simulink model "QD2_MissionCtrl_Hover_FreqSwp_2021a"  (R2026a)
settings: Solver=ode2  StopTime=inf  FixedStep=0.001  EnableMultiTasking=on
undefined symbols (not defined in the file): _MissionCtrl, datetime, Host, log_, m, qc_get_step_size, saved_data
libraries: quarc_library x29, simulink x11, simulink_extras x1
(part 1 of 2)
settings Model: SimulationMode=external  ExtModeTrigDuration=10000  Creator=Admin  LastModifiedBy=jayca
settings SolverCC: PositivePriorityOrder=on
settings RTWCC: SystemTargetFile=quarc_win64.tlc  TemplateMakefile=quarc_default_tmf  Toolchain=QUARC win64 | nmake (64-bit Windows)  BuildConfiguration=Faster Runs  Description=QUARC Win64 Target Using Toolchain
settings STFCustomTargetCC: SystemTargetFile=quarc_win64.tlc  MultiwordLength=2048.0  ConcurrentExecutionCompliant=on  UseToolchainInfoCompliant=on
settings GRTTargetCC: ExtMode=on  ExtModeMexFile=quarc_comm  ExtModeMexArgs='-w -d %d -uri %u -URI_Host tcpip://192.168.2.133:18001'  ParMdlRefBuildCompliant=off  CompOptLevelCompliant=off  CombineOutputUpdateFcns=off  MatFileLogging=off  CPPClassGenCompliant=off  GRTInterface=on

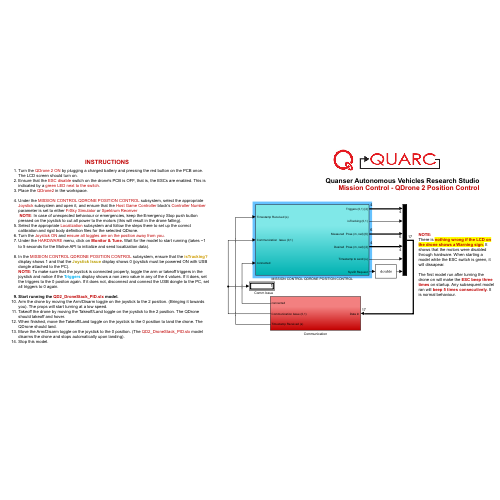
[thumbnail: Simulink's stored preview of the top-level diagram]
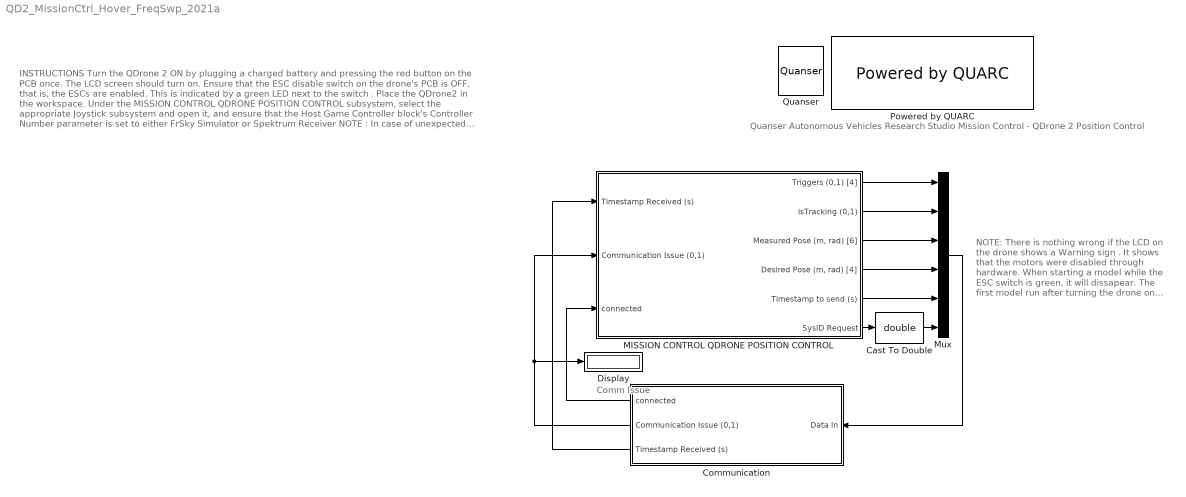
== system QD2_MissionCtrl_Hover_FreqSwp_2021a ==
  note: Quanser Autonomous Vehicles Research Studio
      | Mission Control - QDrone 2 Position Control
  note: Comm Issue
  note: INSTRUCTIONS
      |
      | Turn the QDrone 2 ON by plugging a charged battery and pressing the red button on the PCB once. The LCD screen should turn on.
      | Ensure that the ESC disable switch on the drone's PCB is OFF, that is, the ESCs are enabled. This is indicated by a green LED next to the switch .
      | Place the QDrone2 in the workspace.
      |
      | Under the MISSION CONTROL QDRONE POSITION CONTROL subsystem, select the appropriate Joystick subsystem and open it, and ensure that the Host Game Controller block's Controller Number parameter is set to either FrSky Simulator or Spektrum Receiver
      | NOTE : In case of unexpected behaviour or emergencies, keep the Emergency Stop push button pressed on the joystick to cut all power to the motors (this will result in the drone falling).
      | Select the appropriate Localization subsystem and follow the steps there to set up the correct calibration and rigid body definition files for the selected QDrone.
      | Turn the Joystick ON and ensure all toggles are on the position away from you .
      | Under the HARDWARE menu, click on Monitor & Tune . Wait for the model to start running (takes ~1 to 5 seconds for the Motive API to initialize and send localization data).
      |
      | In the MISSION CONTROL QDRONE POSITION CONTROL subsystem, ensure that the isTracking? display shows 1 and that the Joystick Issue display shows 0 (joystick must be powered ON with USB dongle attached to the PC).
      | NOTE: To make sure that the joystick is connected properly, toggle the arm or takeoff triggers in the joystick and notice if the Triggers display shows a non zero value in any of the 4 values. If it does, set the triggers to the 0 positon again. If it does not, disconnect and connect the USB dongle to the PC, set all triggers to 0 again.
      |
      | Start running the QD2_DroneStack_PID.slx model.
      | Arm the drone by moving the Arm/Disarm toggle on the joystick to the 2 position. (Bringing it towards you). The props will start turning at a low speed.
      | Takeoff the drone by moving the Takeoff/Land toggle on the joystick to the 2 position. The QDrone should takeoff and hover.
      | When finished, move the Takeoff/Land toggle on the joystick to the 0 position to land the drone. The QDrone should land.
      | Move the Arm/Disarm toggle on the joystick to the 0 position. (The QD2_DroneStack_PID.sl x model disarms the drone and stops automatically upon landing).
      | Stop this model.
  note: NOTE:
      | There is nothing wrong if the LCD on the drone shows a Warning sign . It shows that the motors were disabled through hardware. When starting a model while the ESC switch is green, it will dissapear.
      |
      | The first model run after turning the drone on will make the ESC beep three times on startup. Any subsequent model ran will beep 5 times consecutively. It is normal behaviour.
  Cast To Double : DataTypeConversion  OutDataTypeStr=double  SaturateOnIntegerOverflow=off  RndMeth=Floor
  Communication : Subsystem
  Display : Display
  MISSION CONTROL QDRONE POSITION CONTROL : Subsystem
  Mux : Mux  Inputs=6
  Powered by QUARC : quarc_library/Logos/Powered by QUARC
  Quanser : quarc_library/Logos/Quanser
  wires:
  Communication/3(Timestamp Received (s)) -> MISSION CONTROL QDRONE POSITION CONTROL/1(Timestamp Received (s))
  MISSION CONTROL QDRONE POSITION CONTROL/5(Timestamp to send (s)) -> Mux/5
  Mux/1 -> Communication/1(Data In)
  Communication/2(Communication Issue (0,1)) -> MISSION CONTROL QDRONE POSITION CONTROL/2(Communication Issue (0,1)), Display/1
  MISSION CONTROL QDRONE POSITION CONTROL/3("Measured Pose (m, rad) [6]") -> Mux/3
  MISSION CONTROL QDRONE POSITION CONTROL/4("Desired Pose (m, rad) [4]") -> Mux/4
  MISSION CONTROL QDRONE POSITION CONTROL/1(Triggers (0,1) [4]) -> Mux/1
  MISSION CONTROL QDRONE POSITION CONTROL/2(isTracking (0,1)) -> Mux/2
  Communication/1(connected) -> MISSION CONTROL QDRONE POSITION CONTROL/3(connected)
  MISSION CONTROL QDRONE POSITION CONTROL/6(SysID Request) -> Cast To Double/1
  Cast To Double/1 -> Mux/6

== system QD2_MissionCtrl_Hover_FreqSwp_2021a/Communication ==
  note: Argument (-URI_Host) is set at the MEX-file arguments
      | found at Model Configuration Properties > Code Generation > Interface
      |
      | Format:
      | tcpip://localhost:18001
  Data In : Inport
  Compare To Constant : simulink/Logic and Bit Operations/Compare To Constant  relop===  const=2  OutDataTypeStr=boolean
  Constant : Constant
  Detect Communication loss : Subsystem
  Model Argument : quarc_library/Sources/Signals/Model Argument  argument_name=URI_Host  has_value=on  data_type_mode=Specify via dialog  data_type=char  max_length=80  default_value=0  variable_size=off
      settings: AttributesFormatString=(-%<argument_name>)  SourceProductName=QUARC Targets
  Stream Server : quarc_library/Communications/Basic/Stream Server  uri_source=External input port  uri=tcpip://localhost:18877  send_buffer_size=1460  receive_buffer_size=1460  byte_order=little endian (Intel - LSB first)  optimization=Minimum latency  send_options=Send most recent data  receive_options=Receive most recent data  default_value=zeros(1,1)  sample_time=qc_get_step_size  active=off  implementation=Use blocking I/O in a separate thread  send_fifo_size=1000  receive_fifo_size=1000  send_priority=0  receive_priority=0  send_dimensions=off  receive_dimensions=off  max_dimensions=-1  data_type=Inherited via back propagation  type_expr=BusObject
  "String Display " : quarc_library/Strings/String Display  alignment=center  display_mode=Single line  sample_time=-1  use_new=off
      settings: SourceProductName=QUARC Targets
  Terminator1 : Terminator
  Terminator2 : Terminator
  connected : Outport
  Communication Issue (0,1) : Outport  Port=2  VectorParamsAs1DForOutWhenUnconnected=off
  Timestamp Received (s) : Outport  Port=3  VectorParamsAs1DForOutWhenUnconnected=off
  wires:
  Constant/1 -> Stream Server/2
  Data In/1 -> Stream Server/1
  Stream Server/3 -> Terminator2/1
  Stream Server/5 -> Terminator1/1
  Model Argument/1 -> "String Display "/1, Stream Server/3
  Stream Server/4 -> Timestamp Received (s)/1
  Stream Server/2 -> Detect Communication loss/2(Error)
  Detect Communication loss/1(Communication Issue (0,1)) -> Communication Issue (0,1)/1
  Stream Server/1 -> Compare To Constant/1, Detect Communication loss/1(State)
  Compare To Constant/1 -> connected/1

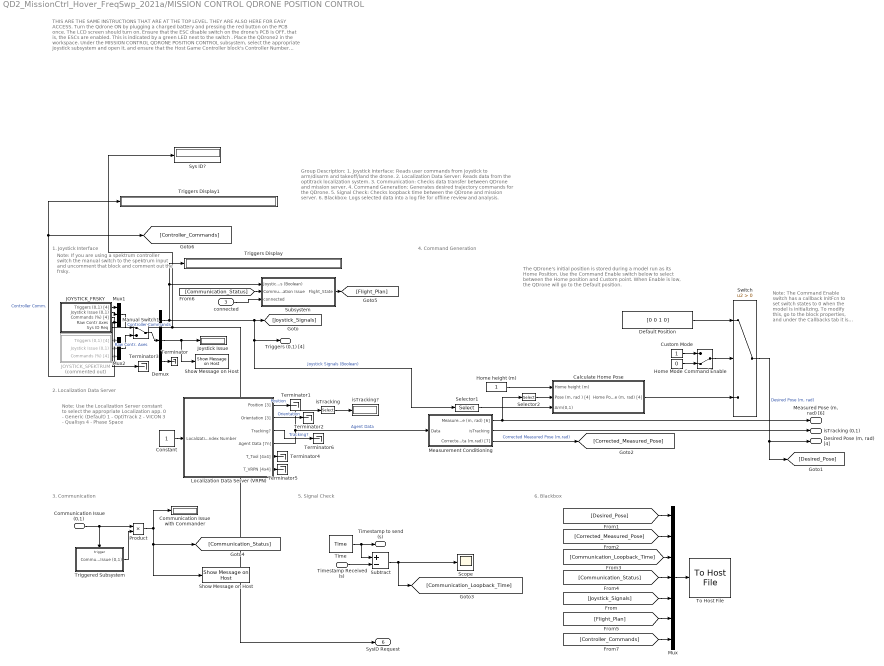
== system QD2_MissionCtrl_Hover_FreqSwp_2021a/MISSION CONTROL QDRONE POSITION CONTROL ==
  note: 5. Signal Check
  note: 6. Blackbox
  note: 3. Communication
  note: 2. Localization Data Server
  note: 1. Joystick Interface
  note: 4. Command Generation
  note: Group Description:
      |
      | 1. Joystick Interface: Reads user commands from joystick to arm/disarm and takeoff/land the drone.
      | 2. Localization Data Server: Reads data from the optitrack localization system.
      | 3. Communication: Checks data transfer between QDrone and mission server.
      | 4. Command Generation: Generates desired trajectory commands for the QDrone.
      | 5. Signal Check: Checks loopback time between the QDrone and mission server.
      | 6. Blackbox: Logs selected data into a log file for offline review and analysis.
  note: THIS ARE THE SAME INSTRUCTIONS THAT ARE AT THE TOP LEVEL. THEY ARE ALSO HERE FOR EASY ACCESS.
      |
      | Turn the Qdrone ON by plugging a charged battery and pressing the red button on the PCB once. The LCD screen should turn on.
      | Ensure that the ESC disable switch on the drone's PCB is OFF, that is, the ESCs are enabled. This is indicated by a green LED next to the switch .
      | Place the QDrone2 in the workspace.
      | Under the MISSION CONTROL QDRONE POSITION CONTROL subsystem, select the appropriate Joystick subsystem and open it, and ensure that the Host Game Controller block's Controller Number parameter is set to either FrSky Simulator or Spektrum Receiver
      | NOTE : In case of unexpected behaviour or emergencies, keep the Emergency Stop push button pressed on the joystick to cut all power to the motors (this will result in the drone falling).
      | Select the appropriate Localization subsystem and follow the steps there to set up the correct calibration and rigid body definition files for the selected QDrone.
      | Turn the Joystick ON and ensure all toggles are on the position away from you .
      | Under the HARDWARE menu, click on Monitor & Tune . Wait for the model to start running (takes ~1 to 5 seconds for the Motive API to initialize and send localization data).
      | In the MISSION CONTROL QDRONE POSITION CONTROL subsystem, ensure that the isTracking? display shows 1 and that the Joystick Issue display shows 0 (joystick must be powered ON with USB dongle attached to the PC).
      | NOTE: To make sure that the joystick is connected properly, toggle the arm or takeoff triggers in the joystick and notice if the Triggers display shows a non zero value in any of the 4 values. If it does, set the triggers to the 0 positon again. If it does not, disconnect and connect the USB dongle to the PC, set all triggers to 0 again.
      | Start running the QD2_DroneStack_PID.slx model.
      | Arm the drone by moving the Arm/Disarm toggle on the joystick to the 2 position. (Bringing it towards you). The props will start turning at a low speed.
      | Takeoff the drone by moving the Takeoff/Land toggle on the joystick to the 2 position. The QDrone should takeoff and hover.
      | When finished, move the Takeoff/Land toggle on the joystick to the 0 position to land the drone. The QDrone should land.
      | Move the Arm/Disarm toggle on the joystick to the 0 position. (The QD2_DroneStack_PID.slx model disarms the drone and stops automatically upon landing).
      | Stop this model.
  note: The QDrone's initial position is stored during a model run as its Home Position.
      | Use the Command Enable switch below to select between the Home position and Custom point. When Enable is low, the QDrone will go to the Default position.
  note: Note:
      | The Command Enable switch has a callback InitFcn to set switch states to 0 when the model is initializing. To modify this, go to the block properties, and under the Callbacks tab it is set in the InitFcn.
  note: Note:
      | If you are using a spektrum controller switch the manual switch to the spektrum input and uncomment that block and comment out the frsky.
  note: Note:
      | Use the Localization Server constant to select the appropriate Localization app.
      |
      | 0 - Generic (Default)
      | 1 - OptiTrack
      | 2 - VICON
      | 3 - Qualisys
      | 4 - Phase Space
  Timestamp Received (s) : Inport
  Communication Issue (0,1) : Inport  Port=2
  connected : Inport  Port=3
  Calculate Home Pose : Subsystem
  Command Enable : ManualSwitch  InitFcn=set_param(gcb,'sw','0')  CurrentSetting=0
  Communication Issue with Commander : Display
  Constant : Constant
  Custom Mode : Constant
  Default Position : Constant  Value=[0 0 1 0]
  Demux : Demux  Outputs=[4 1 4]
  Home Mode : Constant  Value=0
  Home height (m) : Constant
  JOYSTICK_FRSKY : Subsystem
      mask Display: image('$imagefile'); % Use "Edit Image" on toolstrip to change.
  JOYSTICK_SPEKTRUM : Subsystem  Commented=on
      mask Display: image('$imagefile'); % Use "Edit Image" on toolstrip to change.
  Joystick Issue : Display
  "Localization Data Server (VRPN) " : Subsystem
  Manual Switch1 : ManualSwitch
  Measurement Conditioning : Subsystem
  Mux : Mux  Inputs=7
  Mux1 : Mux  Inputs=[4 1 4]
  Mux2 : Mux  Inputs=[4 1 4]
  Product : Product
  Scope : Scope
      settings: ActiveDisplayYMinimum=109.87009  ActiveDisplayYMaximum=111.26511
  Selector1 : Selector  InputPortWidth=4  IndexOptions=Index vector (dialog)  Indices=[1]  OutputSizes=1
  Selector2 : Selector  InputPortWidth=6  IndexOptions=Index vector (dialog)  Indices=[1:3,6]  OutputSizes=1
  Show Message on Host : quarc_library/Sinks/Error Handling/Show Message on Host  message_type=Fixed error message  message_icon=Warning  message=Mission Control: No communication with QDrone
      settings: AttributesFormatString="\"%<message>\""  SourceProductName=QUARC Targets
  "Show Message on Host " : quarc_library/Sinks/Error Handling/Show Message on Host  message_type=Fixed error message  message_icon=Warning  message=Mission Control: Joystick Disconnected
      settings: AttributesFormatString="\"%<message>\""  SourceProductName=QUARC Targets
  Subsystem : Subsystem
  Subtract : Sum  Inputs=+-
  Switch : Switch  Criteria=u2 > Threshold  SaturateOnIntegerOverflow=off  InputSameDT=off
  Sys ID? : Display
  Terminator{,1..6} (7 alike) : Terminator
  Time : quarc_library/Sources/Time/Time  time_source=Wall clock  sample_time=qc_get_step_size
  To Host File : quarc_library/Sinks/To Host/To Host File  source=Specify via dialog (do not evaluate)  file_name=saved_data/%m/log_%{regexprep(char(datetime),' ','_')}_MissionCtrl.mat  variable_name=mission_server_data  decimation=1  sample_time=-1  file_format=MAT-file v.5  options=No header or footer  append=off  final_file_name=saved_data/QD2_MissionCtrl_Hover_FreqSwp_2021a/log_2026-09-15_19-51-03_MissionCtrl.mat  encoding=Default  bitrate=2000000
  Triggered Subsystem : Subsystem  TreatAsAtomicUnit=on
  Triggers Display : Display
  Triggers Display1 : Display
  isTracking : Selector  InputPortWidth=7  IndexOptions=Index vector (dialog)  Indices=[7]  OutputSizes=1
  isTracking? : Display
  Triggers (0,1) [4] : Outport  VectorParamsAs1DForOutWhenUnconnected=off
  isTracking (0,1) : Outport  Port=2  VectorParamsAs1DForOutWhenUnconnected=off
  "Measured Pose (m, rad) [6]" : Outport  Port=3  VectorParamsAs1DForOutWhenUnconnected=off
  "Desired Pose (m, rad) [4]" : Outport  Port=4  VectorParamsAs1DForOutWhenUnconnected=off
  Timestamp to send (s) : Outport  Port=5  VectorParamsAs1DForOutWhenUnconnected=off
  SysID Request : Outport  Port=6
  wires:
  Communication Issue (0,1)/1 -> Product/1, Triggered Subsystem/Trigger
  isTracking/1 -> isTracking?/1
  Demux/2 -> "Show Message on Host "/1, Joystick Issue/1
  Demux/3 -> Terminator/1
  Demux/1 -> Subsystem/1(Joystick Signals (Boolean)), Triggers Display/1, Selector1/1, Triggers (0,1) [4]/1, [Joystick_Signals]  "Joystick Signals (Boolean)"
  Time/1 -> Subtract/1, Timestamp to send (s)/1
  Timestamp Received (s)/1 -> Subtract/2
  Subtract/1 -> Scope/1, [Communication_Loopback_Time]
  Switch/1 -> [Desired_Pose], "Desired Pose (m, rad) [4]"/1  "Desired Pose (m, rad)"
  Measurement Conditioning/2(isTracking) -> isTracking (0,1)/1
  Calculate Home Pose/1("Home Pose (m, rad) [4]") -> Switch/3
  Home height (m)/1 -> Calculate Home Pose/1(Home height (m))
  Triggered Subsystem/1(Communication Issue (0,1)) -> Product/2
  Mux/1 -> To Host File/1
  Selector1/1 -> Calculate Home Pose/3(Arm(0,1))
  Measurement Conditioning/1("Measured Pose (m, rad) [6]") -> "Measured Pose (m, rad) [6]"/1, Selector2/1
  Measurement Conditioning/3(Corrected Pose Data (m,rad) [7]) -> [Corrected_Measured_Pose]  "Corrected Measured Pose (m,rad)"
  JOYSTICK_SPEKTRUM/1(Triggers (0,1) [4]) -> Mux2/1
  JOYSTICK_SPEKTRUM/2(Joystick Issue (0,1)) -> Mux2/2
  JOYSTICK_SPEKTRUM/3(Commands (%) [4]) -> Mux2/3
  Manual Switch1/1 -> Demux/1
  Mux2/1 -> Manual Switch1/2
  Home Mode/1 -> Command Enable/2
  Custom Mode/1 -> Command Enable/1
  Command Enable/1 -> Switch/2
  JOYSTICK_FRSKY/2(Joystick Issue (0,1)) -> Mux1/2
  JOYSTICK_FRSKY/1(Triggers (0,1) [4]) -> Mux1/1
  JOYSTICK_FRSKY/3(Commands (%) [4]) -> Triggers Display1/1, [Controller_Commands], Mux1/3  "Controller Comm."
  Mux1/1 -> Manual Switch1/1  "Controller Commands"
  "Localization Data Server (VRPN) "/4(Agent Data [7n]) -> isTracking/1, Measurement Conditioning/1(Data)  "Agent Data"
  Selector2/1 -> Calculate Home Pose/2("Pose (m, rad ) [4]")
  [Joystick_Signals] -> Mux/5
  [Desired_Pose] -> Mux/1
  [Corrected_Measured_Pose] -> Mux/2
  [Communication_Loopback_Time] -> Mux/3
  [Communication_Status] -> Mux/4
  Subsystem/1(Flight_State) -> [Flight_Plan]
  [Flight_Plan] -> Mux/6
  [Communication_Status] -> Subsystem/2("Communication Issue ")
  Product/1 -> Communication Issue with Commander/1, [Communication_Status], Show Message on Host/1
  Default Position/1 -> Switch/1
  connected/1 -> Subsystem/3(connected)
  Constant/1 -> "Localization Data Server (VRPN) "/1(Localization System Index Number)
  "Localization Data Server (VRPN) "/5(T_Tool [4x4]) -> Terminator4/1
  "Localization Data Server (VRPN) "/6(T_VRPN [4x4]) -> Terminator5/1
  [Controller_Commands] -> Mux/7
  "Localization Data Server (VRPN) "/1(Position [3]) -> Terminator1/1  "Position"
  "Localization Data Server (VRPN) "/2(Orientation [3]) -> Terminator2/1  "Orientation"
  "Localization Data Server (VRPN) "/3(Tracking?) -> Terminator6/1  "Tracking?"
  JOYSTICK_FRSKY/4(Raw Contr Axes) -> Terminator3/1  "Raw Contr. Axes"
  JOYSTICK_FRSKY/5(Sys ID Req) -> Sys ID?/1, SysID Request/1

== system QD2_MissionCtrl_Hover_FreqSwp_2021a/Communication/Detect Communication loss ==
  note: Check if stream is 2 (connected) and error is positive (error codes are negative). Otherwise issue a communication error.
  State : Inport
  Error : Inport  Port=2
  Data Type Conversion : DataTypeConversion  SaturateOnIntegerOverflow=off  RndMeth=Floor
  MATLAB Function : MATLAB Function  TreatAsAtomicUnit=on
  Terminator2 : Terminator
  Threshold : quarc_library/Discontinuities/Threshold  operator=>=  param_src=Specify via dialog  threshold=0.5  duration=0.1
      settings: SourceProductName=QUARC Targets
  Time : quarc_library/Sources/Time/Time  time_source=Wall clock  sample_time=qc_get_step_size
  Communication Issue (0,1) : Outport  VectorParamsAs1DForOutWhenUnconnected=off
  wires:
  Error/1 -> MATLAB Function/3(error)
  MATLAB Function/1(stream_connection_loss) -> Threshold/1
  State/1 -> MATLAB Function/2(state)
  Time/1 -> MATLAB Function/1(time)
  Threshold/2 -> Terminator2/1
  Data Type Conversion/1 -> Communication Issue (0,1)/1
  Threshold/1 -> Data Type Conversion/1

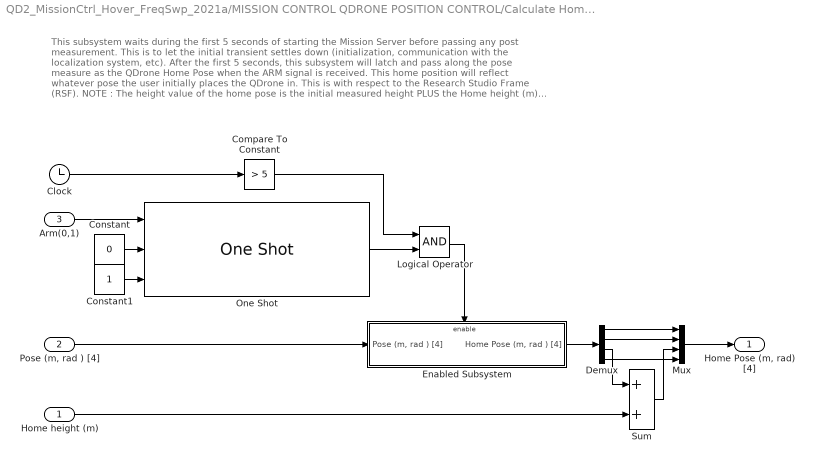
== system QD2_MissionCtrl_Hover_FreqSwp_2021a/MISSION CONTROL QDRONE POSITION CONTROL/Calculate Home Pose ==
  note: This subsystem waits during the first 5 seconds of starting the Mission Server before passing any post measurement.
      | This is to let the initial transient settles down (initialization, communication with the localization system, etc).
      | After the first 5 seconds, this subsystem will latch and pass along the pose measure as the QDrone Home Pose when
      | the ARM signal is received.
      | This home position will reflect whatever pose the user initially places the QDrone in.
      | This is with respect to the Research Studio Frame (RSF).
      |
      | NOTE : The height value of the home pose is the initial measured height PLUS the Home height (m) input value.
  Home height (m) : Inport
  "Pose (m, rad ) [4]" : Inport  Port=2
  Arm(0,1) : Inport  Port=3
  Clock : Clock
  Compare To Constant : simulink/Logic and Bit Operations/Compare To Constant  relop=>  const=5  OutDataTypeStr=boolean
  Constant : Constant  Value=0
  Constant1 : Constant
  Demux : Demux
  Enabled Subsystem : Subsystem  TreatAsAtomicUnit=on
  Logical Operator : Logic  AllPortsSameDT=off  OutDataTypeStr=boolean
  Mux : Mux
  One Shot : quarc_library/Discontinuities/One Shot  trigger_type=Rising edge  redun_pulse=Ignore extraneous pulse  width_source=Specify via dialog  pulse_width=1/qc_get_step_size
      settings: SourceProductName=QUARC Targets
  Sum : Sum
  "Home Pose (m, rad) [4]" : Outport  VectorParamsAs1DForOutWhenUnconnected=off
  wires:
  Constant/1 -> One Shot/2
  Constant1/1 -> One Shot/3
  Arm(0,1)/1 -> One Shot/1
  One Shot/1 -> Logical Operator/2
  "Pose (m, rad ) [4]"/1 -> Enabled Subsystem/1("Pose (m, rad ) [4] ")
  Clock/1 -> Compare To Constant/1
  Compare To Constant/1 -> Logical Operator/1
  Logical Operator/1 -> Enabled Subsystem/Enable
  Enabled Subsystem/1("Home Pose (m, rad ) [4]") -> Demux/1
  Demux/1 -> Mux/1
  Demux/2 -> Mux/2
  Demux/4 -> Mux/4
  Demux/3 -> Sum/1
  Sum/1 -> Mux/3
  Home height (m)/1 -> Sum/2
  Mux/1 -> "Home Pose (m, rad) [4]"/1

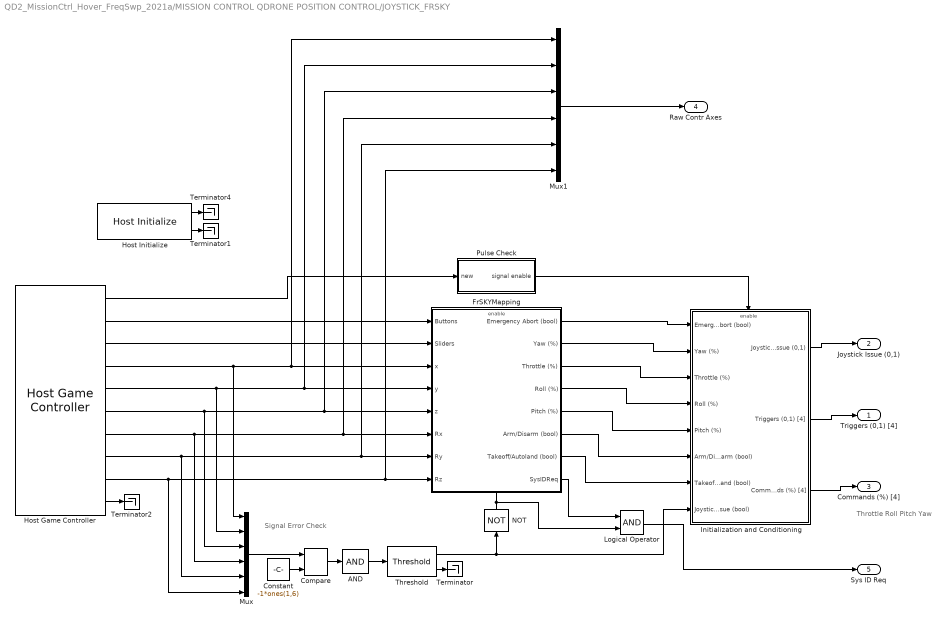
== system QD2_MissionCtrl_Hover_FreqSwp_2021a/MISSION CONTROL QDRONE POSITION CONTROL/JOYSTICK_FRSKY ==
  note: Throttle
      | Roll
      | Pitch
      | Yaw
  note: Signal Error Check
  AND : Logic  Inputs=1  AllPortsSameDT=off  OutDataTypeStr=boolean
  Compare : quarc_library/Logic Operations/Compare  operator===  output_data_type=boolean
      settings: SourceProductName=QUARC Targets
  Constant : Constant  Value=-1*ones(1,6)
  FrSKYMapping : Subsystem
  Host Game Controller : quarc_library/Devices/Peripherals/Host/Host Game Controller  object_name=Host-1  controller=1  buffer_size=20  deadzone=[]  saturation=[]  sample_time=qc_get_step_size  auto_center=off  enabled=on  debug_mode=off
      settings: SourceProductName=QUARC Targets
  Host Initialize : quarc_library/Devices/Peripherals/Host/Host Initialize  object_name=Host-1  uri_source=Use external mode communications  uri=tcpip://localhost:18001  send_buffer_size=1000  receive_buffer_size=1000  thread_priority=0  run_client=on  use_window=off  window_position=[]  sample_time=qc_get_step_size  active=on
      settings: SourceProductName=QUARC Targets
  Initialization and Conditioning : Subsystem  TreatAsAtomicUnit=on
  Logical Operator : Logic  AllPortsSameDT=off  OutDataTypeStr=boolean
  Mux : Mux  Inputs=6
  Mux1 : Mux  Inputs=6
  NOT : Logic  Operator=NOT  IconShape=distinctive  AllPortsSameDT=off  OutDataTypeStr=boolean
  Pulse Check : Subsystem  TreatAsAtomicUnit=on
  Terminator{,1..2,4} (4 alike) : Terminator
  Threshold : quarc_library/Discontinuities/Threshold  operator=>=  param_src=Specify via dialog  threshold=0.5  duration=0.2
      settings: SourceProductName=QUARC Targets
  Triggers (0,1) [4] : Outport  VectorParamsAs1DForOutWhenUnconnected=off
  Joystick Issue (0,1) : Outport  Port=2  VectorParamsAs1DForOutWhenUnconnected=off
  Commands (%) [4] : Outport  Port=3  VectorParamsAs1DForOutWhenUnconnected=off
  Raw Contr Axes : Outport  Port=4
  Sys ID Req : Outport  Port=5
  wires:
  Host Game Controller/10 -> Terminator2/1
  Pulse Check/1(signal enable) -> Initialization and Conditioning/Enable
  Host Initialize/1 -> Terminator4/1
  FrSKYMapping/6("Arm/Disarm (bool) ") -> Initialization and Conditioning/6(Arm/Disarm (bool))
  Host Initialize/2 -> Terminator1/1
  FrSKYMapping/7(Takeoff/Autoland (bool)) -> Initialization and Conditioning/7(Takeoff/AutoLand (bool))
  Host Game Controller/7 -> Mux/4, Mux1/4, FrSKYMapping/6(Rx)
  Host Game Controller/8 -> Mux/5, Mux1/5, FrSKYMapping/7(Ry)
  Initialization and Conditioning/3(Commands (%) [4]) -> Commands (%) [4]/1
  Host Game Controller/5 -> Mux/2, Mux1/2, FrSKYMapping/4(y)
  Host Game Controller/9 -> Mux/6, Mux1/6, FrSKYMapping/8(Rz)
  Host Game Controller/1 -> Pulse Check/1(new)
  Mux/1 -> Compare/1
  Threshold/1 -> NOT/1, Initialization and Conditioning/8(Joystick Issue (bool))
  AND/1 -> Threshold/1
  Host Game Controller/3 -> FrSKYMapping/2(Sliders)
  Threshold/2 -> Terminator/1
  NOT/1 -> Logical Operator/2, FrSKYMapping/Enable
  Constant/1 -> Compare/2
  Host Game Controller/6 -> Mux/3, Mux1/3, FrSKYMapping/5(z)
  FrSKYMapping/4(Roll (%)) -> Initialization and Conditioning/4(Roll (%))
  FrSKYMapping/5(Pitch (%)) -> Initialization and Conditioning/5(Pitch (%))
  Compare/1 -> AND/1
  Initialization and Conditioning/1(Joystick Issue (0,1)) -> Joystick Issue (0,1)/1
  Initialization and Conditioning/2(Triggers (0,1) [4]) -> Triggers (0,1) [4]/1
  FrSKYMapping/2(Yaw (%)) -> Initialization and Conditioning/2(Yaw (%))
  Host Game Controller/4 -> Mux1/1, FrSKYMapping/3(x), Mux/1
  Host Game Controller/2 -> FrSKYMapping/1(Buttons)
  FrSKYMapping/3(Throttle (%)) -> Initialization and Conditioning/3(Throttle (%))
  Mux1/1 -> Raw Contr Axes/1
  FrSKYMapping/1(Emergency Abort (bool)) -> Initialization and Conditioning/1(Emergency Abort (bool))
  FrSKYMapping/8(SysIDReq) -> Logical Operator/1
  Logical Operator/1 -> Sys ID Req/1

== system QD2_MissionCtrl_Hover_FreqSwp_2021a/MISSION CONTROL QDRONE POSITION CONTROL/JOYSTICK_SPEKTRUM ==
  note: Throttle
      | Roll
      | Pitch
      | Yaw
  Host Game Controller : quarc_library/Devices/Peripherals/Host/Host Game Controller  object_name=Host-2  controller=1  buffer_size=20  deadzone=[]  saturation=[]  sample_time=qc_get_step_size  auto_center=off  enabled=on  debug_mode=off
      settings: SourceProductName=QUARC Targets
  Host Initialize : quarc_library/Devices/Peripherals/Host/Host Initialize  object_name=Host-2  uri_source=Use external mode communications  uri=tcpip://localhost:18001  send_buffer_size=1000  receive_buffer_size=1000  thread_priority=0  run_client=on  use_window=off  window_position=[]  sample_time=qc_get_step_size  active=on
      settings: SourceProductName=QUARC Targets
  Initialization and Conditioning : Subsystem  TreatAsAtomicUnit=on
  Pulse Check : Subsystem  TreatAsAtomicUnit=on
  Spectrum DXe Mapping : Subsystem
  Terminator{1..4} (4 alike) : Terminator
  Triggers (0,1) [4] : Outport  VectorParamsAs1DForOutWhenUnconnected=off
  Joystick Issue (0,1) : Outport  Port=2  VectorParamsAs1DForOutWhenUnconnected=off
  Commands (%) [4] : Outport  Port=3  VectorParamsAs1DForOutWhenUnconnected=off
  wires:
  Pulse Check/1(signal enable) -> Initialization and Conditioning/Enable
  Host Game Controller/1 -> Pulse Check/1(new), Spectrum DXe Mapping/1(new)
  Initialization and Conditioning/3(Commands (%) [4]) -> Commands (%) [4]/1
  Spectrum DXe Mapping/8(Takeoff/Autoland (bool)) -> Initialization and Conditioning/8(Takeoff/AutoLand (bool))
  Initialization and Conditioning/2(Triggers (0,1) [4]) -> Triggers (0,1) [4]/1
  Spectrum DXe Mapping/2(Emergency Abort (bool)) -> Initialization and Conditioning/2(Emergency Abort (bool))
  Host Game Controller/2 -> Spectrum DXe Mapping/2(buttons)
  Spectrum DXe Mapping/6(Pitch (%)) -> Initialization and Conditioning/6(Pitch (%))
  Spectrum DXe Mapping/4(Throttle (%)) -> Initialization and Conditioning/4(Throttle (%))
  Spectrum DXe Mapping/5(Roll (%)) -> Initialization and Conditioning/5(Roll (%))
  Spectrum DXe Mapping/7("Arm/Disarm (bool) ") -> Initialization and Conditioning/7(Arm/Disarm (bool))
  Spectrum DXe Mapping/3(Yaw (%)) -> Initialization and Conditioning/3(Yaw (%))
  Host Initialize/2 -> Terminator1/1
  Host Initialize/1 -> Terminator4/1
  Host Game Controller/6 -> Spectrum DXe Mapping/6(z)
  Host Game Controller/3 -> Spectrum DXe Mapping/3(Sliders)
  Host Game Controller/5 -> Spectrum DXe Mapping/5(y)
  Host Game Controller/4 -> Spectrum DXe Mapping/4(x)
  Host Game Controller/8 -> Spectrum DXe Mapping/8(Ry)
  Host Game Controller/9 -> Terminator2/1
  Host Game Controller/10 -> Terminator3/1
  Host Game Controller/7 -> Spectrum DXe Mapping/7(Rx)
  Spectrum DXe Mapping/1(Joystick Issue (bool)) -> Initialization and Conditioning/1(Joystick Issue (bool))
  Initialization and Conditioning/1(Joystick Issue (0,1)) -> Joystick Issue (0,1)/1

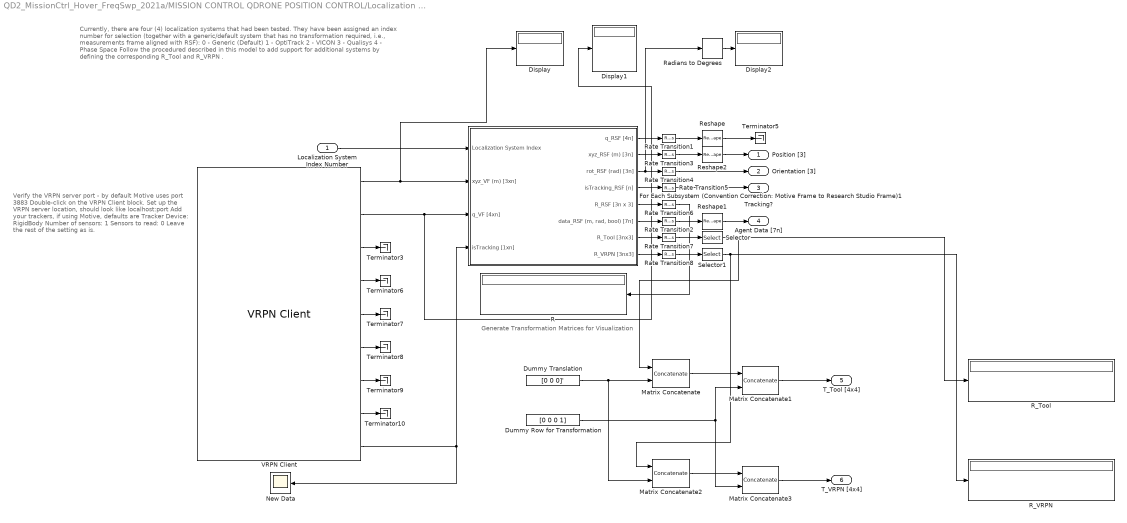
== system QD2_MissionCtrl_Hover_FreqSwp_2021a/MISSION CONTROL QDRONE POSITION CONTROL/Localization Data Server (VRPN)  ==
  note: Currently, there are four (4) localization systems that had been tested. They have been assigned an index number for selection (together with a generic/default system that has no transformation required, i.e., measurements frame aligned with RSF):
      |
      | 0 - Generic (Default)
      | 1 - OptiTrack
      | 2 - VICON
      | 3 - Qualisys
      | 4 - Phase Space
      |
      | Follow the procedured described in this model to add support for additional systems by defining the corresponding R_Tool and R_VRPN .
  note: Verify the VRPN server port - by default Motive uses port 3883
      | Double-click on the VRPN Client block.
      |
      | Set up the VRPN server location, should look like
      | localhost:port
      |
      | Add your trackers,
      | if using Motive, defaults are
      | Tracker Device: RigidBody
      | Number of sensors: 1
      | Sensors to read: 0
      |
      | Leave the rest of the setting as is.
  note: Generate Transformation Matrices for Visualization
  Localization System Index Number : Inport
  Display : Display
  Display1 : Display
  Display2 : Display
  Dummy Row for Transformation : Constant  Value=[0 0 0 1]  VectorParams1D=off
  Dummy Translation : Constant  Value=[0 0 0]'  VectorParams1D=off
  For Each Subsystem (Convention Correction: Motive Frame to Research Studio Frame)1 : Subsystem  TreatAsAtomicUnit=on
  Matrix Concatenate : Concatenate  Mode=Multidimensional array  ConcatenateDimension=2
  Matrix Concatenate1 : Concatenate  Mode=Multidimensional array
  Matrix Concatenate2 : Concatenate  Mode=Multidimensional array  ConcatenateDimension=2
  Matrix Concatenate3 : Concatenate  Mode=Multidimensional array
  New Data : Scope
      settings: ActiveDisplayYMinimum=-1  ActiveDisplayYMaximum=1
  R : Display
  R_Tool : Display
  R_VRPN : Display
  Radians to Degrees : simulink_extras/Transformations/Radians to Degrees
  Rate Transition{1..8} (8 alike) : RateTransition
  Reshape : Reshape
  Reshape1 : Reshape
  Reshape2 : Reshape
  Selector : Selector  NumberOfDimensions=2  InputPortWidth=3  IndexOptions=Index vector (dialog),Index vector (dialog)  Indices=[1:3],[1:3]  OutputSizes=1,1
  Selector1 : Selector  NumberOfDimensions=2  InputPortWidth=3  IndexOptions=Index vector (dialog),Index vector (dialog)  Indices=[1:3],[1:3]  OutputSizes=1,1
  Terminator{3,5..10} (7 alike) : Terminator
  VRPN Client : quarc_library/Devices/Third-Party/VRPN/VRPN Client  server_address=192.168.2.5:3883  trackerstable={ 'QDrone2_02', '1', '0' }  trackers_list_mask='QDrone2_02'  trackers_num_sensors=[1]  trackers_sensors_to_read_arg="[1  0]"  trackers_jpl=off  sample_time=qc_get_step_size*16  active=on
      settings: SourceProductName=QUARC Targets
  Position [3] : Outport  VectorParamsAs1DForOutWhenUnconnected=off
  Orientation [3] : Outport  Port=2  VectorParamsAs1DForOutWhenUnconnected=off
  Tracking? : Outport  Port=3  VectorParamsAs1DForOutWhenUnconnected=off
  Agent Data [7n] : Outport  Port=4  VectorParamsAs1DForOutWhenUnconnected=off
  T_Tool [4x4] : Outport  Port=5  VectorParamsAs1DForOutWhenUnconnected=off
  T_VRPN [4x4] : Outport  Port=6  VectorParamsAs1DForOutWhenUnconnected=off
  wires:
  Radians to Degrees/1 -> Display2/1
  Matrix Concatenate3/1 -> T_VRPN [4x4]/1
  Selector1/1 -> R_VRPN/1, Matrix Concatenate2/1
  Matrix Concatenate2/1 -> Matrix Concatenate3/1
  Dummy Row for Transformation/1 -> Matrix Concatenate1/2, Matrix Concatenate3/2
  Matrix Concatenate1/1 -> T_Tool [4x4]/1
  Matrix Concatenate/1 -> Matrix Concatenate1/1
  Dummy Translation/1 -> Matrix Concatenate/2, Matrix Concatenate2/2
  Selector/1 -> R_Tool/1, Matrix Concatenate/1
  For Each Subsystem (Convention Correction: Motive Frame to Research Studio Frame)1/8(R_VRPN [3nx3]) -> Rate Transition8/1
  Rate Transition8/1 -> Selector1/1
  Rate Transition7/1 -> Selector/1
  For Each Subsystem (Convention Correction: Motive Frame to Research Studio Frame)1/7(R_Tool [3nx3]) -> Rate Transition7/1
  Localization System Index Number/1 -> For Each Subsystem (Convention Correction: Motive Frame to Research Studio Frame)1/1(Localization System Index)
  Rate Transition6/1 -> R/1
  For Each Subsystem (Convention Correction: Motive Frame to Research Studio Frame)1/5(R_RSF [3n x 3]) -> Rate Transition6/1
  Rate Transition5/1 -> Tracking?/1
  Rate Transition4/1 -> Orientation [3]/1
  Rate Transition3/1 -> Reshape2/1
  Reshape2/1 -> Position [3]/1
  Reshape1/1 -> Agent Data [7n]/1
  Rate Transition1/1 -> Reshape/1
  Rate Transition2/1 -> Reshape1/1
  For Each Subsystem (Convention Correction: Motive Frame to Research Studio Frame)1/1(q_RSF [4n]) -> Rate Transition1/1
  For Each Subsystem (Convention Correction: Motive Frame to Research Studio Frame)1/6("data_RSF (m, rad, bool) [7n]") -> Rate Transition2/1
  VRPN Client/9 -> New Data/1, For Each Subsystem (Convention Correction: Motive Frame to Research Studio Frame)1/4(isTracking [1xn])
  VRPN Client/8 -> Terminator10/1
  VRPN Client/7 -> Terminator9/1
  VRPN Client/6 -> Terminator8/1
  VRPN Client/5 -> Terminator7/1
  VRPN Client/4 -> Terminator6/1
  Reshape/1 -> Terminator5/1
  VRPN Client/3 -> Terminator3/1
  For Each Subsystem (Convention Correction: Motive Frame to Research Studio Frame)1/2(xyz_RSF (m) [3n]) -> Rate Transition3/1
  For Each Subsystem (Convention Correction: Motive Frame to Research Studio Frame)1/3(rot_RSF (rad) [3n]) -> Rate Transition4/1, Radians to Degrees/1
  For Each Subsystem (Convention Correction: Motive Frame to Research Studio Frame)1/4(isTracking_RSF [n]) -> Rate Transition5/1
  VRPN Client/2 -> For Each Subsystem (Convention Correction: Motive Frame to Research Studio Frame)1/3(q_VF [4xn]), Display1/1
  VRPN Client/1 -> For Each Subsystem (Convention Correction: Motive Frame to Research Studio Frame)1/2(xyz_VF (m) [3xn]), Display/1

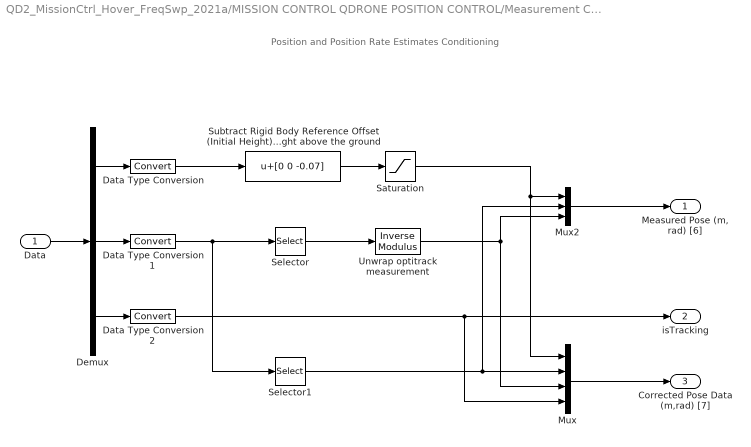
== system QD2_MissionCtrl_Hover_FreqSwp_2021a/MISSION CONTROL QDRONE POSITION CONTROL/Measurement Conditioning ==
  note: Position and Position Rate Estimates Conditioning
  Data : Inport
  Data Type Conversion : DataTypeConversion  SaturateOnIntegerOverflow=off  RndMeth=Floor
  Data Type Conversion1 : DataTypeConversion  SaturateOnIntegerOverflow=off  RndMeth=Floor
  Data Type Conversion2 : DataTypeConversion  SaturateOnIntegerOverflow=off  RndMeth=Floor
  Demux : Demux  Outputs=[3 3 1]
  Mux : Mux
  Mux2 : Mux  Inputs=[3 2 1]
  Saturation : Saturate  UpperLimit=[2 2 5]  LowerLimit=[-2 -2 0]
  Selector : Selector  InputPortWidth=3  IndexOptions=Index vector (dialog)  Indices=[3]  OutputSizes=1
  Selector1 : Selector  InputPortWidth=3  IndexOptions=Index vector (dialog)  Indices=[1 2]  OutputSizes=1
  Subtract Rigid Body Reference Offset (Initial Height) to get height above the ground : Bias  Bias=[0 0 -0.07]  SaturateOnIntegerOverflow=off
  Unwrap optitrack measurement : quarc_library/Discontinuities/Inverse Modulus  modulus=2*pi  output_derivative=off  output_revolutions=off  max_x=Inf  min_x=-Inf
  "Measured Pose (m, rad) [6]" : Outport  VectorParamsAs1DForOutWhenUnconnected=off
  isTracking : Outport  Port=2  VectorParamsAs1DForOutWhenUnconnected=off
  Corrected Pose Data (m,rad) [7] : Outport  Port=3  VectorParamsAs1DForOutWhenUnconnected=off
  wires:
  Demux/2 -> Data Type Conversion1/1
  Demux/1 -> Data Type Conversion/1
  Demux/3 -> Data Type Conversion2/1
  Mux2/1 -> "Measured Pose (m, rad) [6]"/1
  Data/1 -> Demux/1
  Data Type Conversion2/1 -> Mux/4, isTracking/1
  Subtract Rigid Body Reference Offset (Initial Height) to get height above the ground/1 -> Saturation/1
  Saturation/1 -> Mux2/1, Mux/1
  Data Type Conversion1/1 -> Selector1/1, Selector/1
  Selector/1 -> Unwrap optitrack measurement/1
  Data Type Conversion/1 -> Subtract Rigid Body Reference Offset (Initial Height) to get height above the ground/1
  Unwrap optitrack measurement/1 -> Mux2/3, Mux/3
  Mux/1 -> Corrected Pose Data (m,rad) [7]/1
  Selector1/1 -> Mux2/2, Mux/2

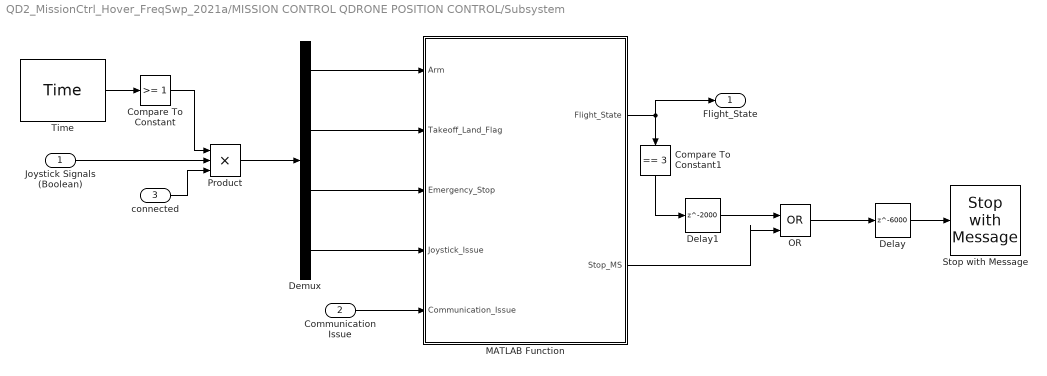
== system QD2_MissionCtrl_Hover_FreqSwp_2021a/MISSION CONTROL QDRONE POSITION CONTROL/Subsystem ==
  Joystick Signals (Boolean) : Inport
  "Communication Issue " : Inport  Port=2
  connected : Inport  Port=3
  Compare To Constant : simulink/Logic and Bit Operations/Compare To Constant  relop=>=  const=1  OutDataTypeStr=boolean
  Compare To Constant1 : simulink/Logic and Bit Operations/Compare To Constant  relop===  const=3  OutDataTypeStr=boolean
  Delay : Delay  DelayLength=6000
  Delay1 : Delay  DelayLength=2000
  Demux : Demux
  MATLAB Function : MATLAB Function  TreatAsAtomicUnit=on
  OR : Logic  Operator=OR  IconShape=distinctive  AllPortsSameDT=off  OutDataTypeStr=boolean
  Product : Product  Inputs=3
  Stop with Message : quarc_library/Sinks/Error Handling/Stop with Message  message_type=Fixed error message  message_icon=Information  message=Mission plan ended, stopping mission control!
  Time : quarc_library/Sources/Time/Time  time_source=Wall clock  sample_time=qc_get_step_size
  Flight_State : Outport
  wires:
  Joystick Signals (Boolean)/1 -> Product/2
  Demux/1 -> MATLAB Function/1(Arm)
  Demux/2 -> MATLAB Function/2(Takeoff_Land_Flag)
  Demux/3 -> MATLAB Function/3(Emergency_Stop)
  Demux/4 -> MATLAB Function/4(Joystick_Issue)
  MATLAB Function/1(Flight_State) -> Flight_State/1, Compare To Constant1/1
  Product/1 -> Demux/1
  Time/1 -> Compare To Constant/1
  Compare To Constant/1 -> Product/1
  Delay/1 -> Stop with Message/1
  MATLAB Function/2(Stop_MS) -> OR/2
  OR/1 -> Delay/1
  Compare To Constant1/1 -> Delay1/1
  "Communication Issue "/1 -> MATLAB Function/5(Communication_Issue)
  connected/1 -> Product/3
  Delay1/1 -> OR/1

== system QD2_MissionCtrl_Hover_FreqSwp_2021a/MISSION CONTROL QDRONE POSITION CONTROL/Triggered Subsystem ==
  note: This looks for the first falling edge of the communication issue before allowing a communication issue to be triggered,
      | because the mission server model starts first.
  Trigger : TriggerPort  TriggerType=falling  VariantControl=Variant
  Add : Sum
  Compare To Constant : simulink/Logic and Bit Operations/Compare To Constant  relop=>=  const=1  OutDataTypeStr=boolean
  Constant : Constant
  Memory : Memory  InheritSampleTime=on
  Communication Issue (0,1) : Outport  InitialOutput=0  VectorParamsAs1DForOutWhenUnconnected=off
  wires:
  Constant/1 -> Add/1
  Memory/1 -> Add/2
  Add/1 -> Compare To Constant/1, Memory/1
  Compare To Constant/1 -> Communication Issue (0,1)/1

== system QD2_MissionCtrl_Hover_FreqSwp_2021a/MISSION CONTROL QDRONE POSITION CONTROL/Calculate Home Pose/Enabled Subsystem ==
  "Pose (m, rad ) [4] " : Inport
  Enable : EnablePort
  "Home Pose (m, rad ) [4]" : Outport  VectorParamsAs1DForOutWhenUnconnected=off
  wires:
  "Pose (m, rad ) [4] "/1 -> "Home Pose (m, rad ) [4]"/1

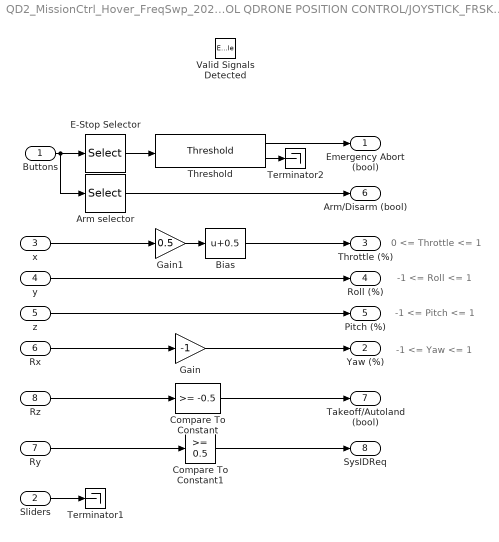
== system QD2_MissionCtrl_Hover_FreqSwp_2021a/MISSION CONTROL QDRONE POSITION CONTROL/JOYSTICK_FRSKY/FrSKYMapping ==
  note: -1 <= Yaw <= 1
  note: 0 <= Throttle <= 1
  note: -1 <= Roll <= 1
  note: -1 <= Pitch <= 1
  Buttons : Inport
  Sliders : Inport  Port=2
  x : Inport  Port=3
  y : Inport  Port=4
  z : Inport  Port=5
  Rx : Inport  Port=6
  Ry : Inport  Port=7
  Rz : Inport  Port=8
  Valid Signals Detected : EnablePort
  Arm selector : Selector  InputPortWidth=32  IndexOptions=Index vector (dialog)  Indices=[2]  OutputSizes=1
  Bias : Bias  Bias=0.5  SaturateOnIntegerOverflow=off
  Compare To Constant : simulink/Logic and Bit Operations/Compare To Constant  relop=>=  const=-0.5  OutDataTypeStr=boolean
  Compare To Constant1 : simulink/Logic and Bit Operations/Compare To Constant  relop=>=  const=0.5  OutDataTypeStr=boolean
  E-Stop Selector : Selector  InputPortWidth=32  IndexOptions=Index vector (dialog)  Indices=[1]  OutputSizes=1
  Gain : Gain  Gain=-1
  Gain1 : Gain  Gain=0.5
  Terminator1 : Terminator
  Terminator2 : Terminator
  Threshold : quarc_library/Discontinuities/Threshold  operator=>=  param_src=Specify via dialog  threshold=0.5  duration=0.2
      settings: SourceProductName=QUARC Targets
  Emergency Abort (bool) : Outport  VectorParamsAs1DForOutWhenUnconnected=off
  Yaw (%) : Outport  Port=2  VectorParamsAs1DForOutWhenUnconnected=off
  Throttle (%) : Outport  Port=3  VectorParamsAs1DForOutWhenUnconnected=off
  Roll (%) : Outport  Port=4  VectorParamsAs1DForOutWhenUnconnected=off
  Pitch (%) : Outport  Port=5  VectorParamsAs1DForOutWhenUnconnected=off
  "Arm/Disarm (bool) " : Outport  Port=6  VectorParamsAs1DForOutWhenUnconnected=off
  Takeoff/Autoland (bool) : Outport  Port=7  VectorParamsAs1DForOutWhenUnconnected=off
  SysIDReq : Outport  Port=8
  wires:
  Buttons/1 -> Arm selector/1, E-Stop Selector/1
  Arm selector/1 -> "Arm/Disarm (bool) "/1
  x/1 -> Gain1/1
  y/1 -> Roll (%)/1
  z/1 -> Pitch (%)/1
  Rx/1 -> Gain/1
  Ry/1 -> Compare To Constant1/1
  Sliders/1 -> Terminator1/1
  E-Stop Selector/1 -> Threshold/1
  Rz/1 -> Compare To Constant/1
  Compare To Constant/1 -> Takeoff/Autoland (bool)/1
  Threshold/1 -> Emergency Abort (bool)/1
  Threshold/2 -> Terminator2/1
  Gain/1 -> Yaw (%)/1
  Gain1/1 -> Bias/1
  Bias/1 -> Throttle (%)/1
  Compare To Constant1/1 -> SysIDReq/1

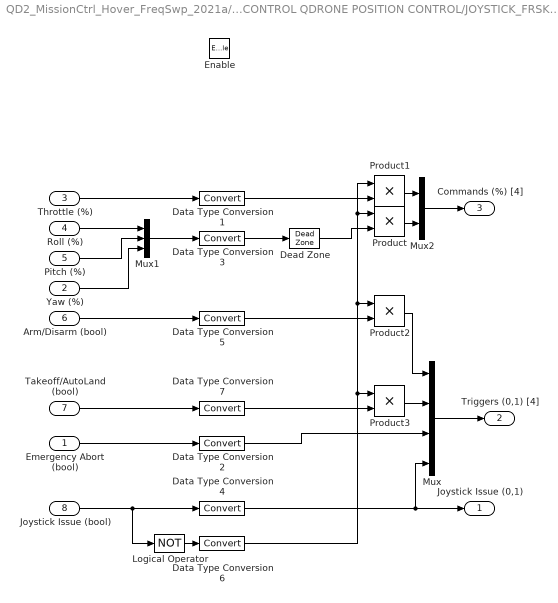
== system QD2_MissionCtrl_Hover_FreqSwp_2021a/MISSION CONTROL QDRONE POSITION CONTROL/JOYSTICK_FRSKY/Initialization and Conditioning ==
  Emergency Abort (bool) : Inport
  Yaw (%) : Inport  Port=2
  Throttle (%) : Inport  Port=3
  Roll (%) : Inport  Port=4
  Pitch (%) : Inport  Port=5
  Arm/Disarm (bool) : Inport  Port=6
  Takeoff/AutoLand (bool) : Inport  Port=7
  Joystick Issue (bool) : Inport  Port=8
  Enable : EnablePort  StatesWhenEnabling=reset
  Data Type Conversion{1..7} (7 alike) : DataTypeConversion  SaturateOnIntegerOverflow=off  RndMeth=Floor
  Dead Zone : DeadZone  LowerValue=-0.01  UpperValue=0.01
  Logical Operator : Logic  Operator=NOT  AllPortsSameDT=off  OutDataTypeStr=boolean
  Mux : Mux
  Mux1 : Mux  Inputs=3
  Mux2 : Mux  Inputs=2
  Product{,1..3} (4 alike) : Product
  Joystick Issue (0,1) : Outport  InitialOutput=0  VectorParamsAs1DForOutWhenUnconnected=off
  Triggers (0,1) [4] : Outport  Port=2  InitialOutput=0  VectorParamsAs1DForOutWhenUnconnected=off
  Commands (%) [4] : Outport  Port=3  InitialOutput=0  VectorParamsAs1DForOutWhenUnconnected=off
  wires:
  Joystick Issue (bool)/1 -> Data Type Conversion4/1, Logical Operator/1
  Mux1/1 -> Data Type Conversion3/1
  Throttle (%)/1 -> Data Type Conversion1/1
  Roll (%)/1 -> Mux1/1
  Pitch (%)/1 -> Mux1/2
  Yaw (%)/1 -> Mux1/3
  Data Type Conversion4/1 -> Mux/4, Joystick Issue (0,1)/1
  Emergency Abort (bool)/1 -> Data Type Conversion2/1
  Data Type Conversion3/1 -> Dead Zone/1
  Arm/Disarm (bool)/1 -> Data Type Conversion5/1
  Mux/1 -> Triggers (0,1) [4]/1
  Data Type Conversion2/1 -> Mux/3
  Logical Operator/1 -> Data Type Conversion6/1
  Product/1 -> Mux2/2
  Product1/1 -> Mux2/1
  Data Type Conversion1/1 -> Product1/2
  Dead Zone/1 -> Product/2
  Data Type Conversion6/1 -> Product1/1, Product/1, Product2/1, Product3/1
  Product2/1 -> Mux/1
  Data Type Conversion5/1 -> Product2/2
  Takeoff/AutoLand (bool)/1 -> Data Type Conversion7/1
  Product3/1 -> Mux/2
  Data Type Conversion7/1 -> Product3/2
  Mux2/1 -> Commands (%) [4]/1

== system QD2_MissionCtrl_Hover_FreqSwp_2021a/MISSION CONTROL QDRONE POSITION CONTROL/JOYSTICK_FRSKY/Pulse Check ==
  note: For this subsystem we will count the number of new pulses. The data can be considered enabled once the count of new signals has gone beyond 2. This will enable the Initializing and conditioning subsystem.
  new : Inport
  Compare : quarc_library/Logic Operations/Compare  operator=>=  output_data_type=boolean
      settings: SourceProductName=QUARC Targets
  Pulse Check : Constant
  "pulse count " : Subsystem  TreatAsAtomicUnit=on
  signal enable : Outport  InitialOutput=0  VectorParamsAs1DForOutWhenUnconnected=off
  wires:
  Compare/1 -> signal enable/1
  Pulse Check/1 -> Compare/2
  new/1 -> "pulse count "/Trigger
  "pulse count "/1(Number of Pulses) -> Compare/1

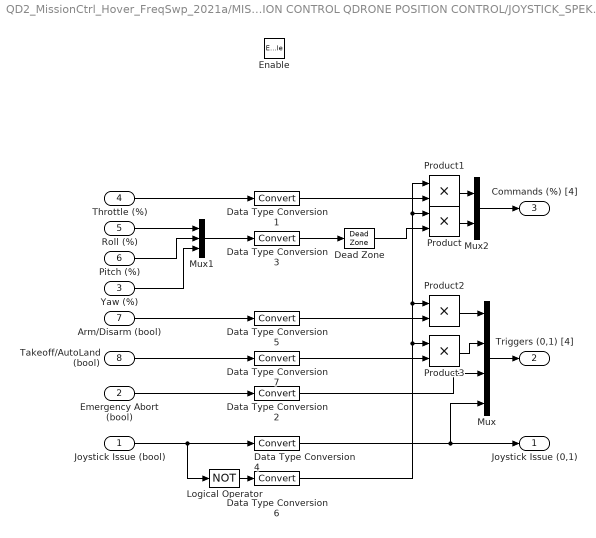
== system QD2_MissionCtrl_Hover_FreqSwp_2021a/MISSION CONTROL QDRONE POSITION CONTROL/JOYSTICK_SPEKTRUM/Initialization and Conditioning ==
  Joystick Issue (bool) : Inport
  Emergency Abort (bool) : Inport  Port=2
  Yaw (%) : Inport  Port=3
  Throttle (%) : Inport  Port=4
  Roll (%) : Inport  Port=5
  Pitch (%) : Inport  Port=6
  Arm/Disarm (bool) : Inport  Port=7
  Takeoff/AutoLand (bool) : Inport  Port=8
  Enable : EnablePort  StatesWhenEnabling=reset
  Data Type Conversion{1..7} (7 alike) : DataTypeConversion  SaturateOnIntegerOverflow=off  RndMeth=Floor
  Dead Zone : DeadZone  LowerValue=-0.01  UpperValue=0.01
  Logical Operator : Logic  Operator=NOT  AllPortsSameDT=off  OutDataTypeStr=boolean
  Mux : Mux
  Mux1 : Mux  Inputs=3
  Mux2 : Mux  Inputs=2
  Product{,1..3} (4 alike) : Product
  Joystick Issue (0,1) : Outport  InitialOutput=0  VectorParamsAs1DForOutWhenUnconnected=off
  Triggers (0,1) [4] : Outport  Port=2  InitialOutput=0  VectorParamsAs1DForOutWhenUnconnected=off
  Commands (%) [4] : Outport  Port=3  InitialOutput=0  VectorParamsAs1DForOutWhenUnconnected=off
  wires:
  Mux2/1 -> Commands (%) [4]/1
  Data Type Conversion7/1 -> Product3/2
  Product3/1 -> Mux/2
  Takeoff/AutoLand (bool)/1 -> Data Type Conversion7/1
  Data Type Conversion5/1 -> Product2/2
  Product2/1 -> Mux/1
  Data Type Conversion6/1 -> Product3/1, Product2/1, Product/1, Product1/1
  Dead Zone/1 -> Product/2
  Data Type Conversion1/1 -> Product1/2
  Product1/1 -> Mux2/1
  Product/1 -> Mux2/2
  Logical Operator/1 -> Data Type Conversion6/1
  Data Type Conversion2/1 -> Mux/3
  Mux/1 -> Triggers (0,1) [4]/1
  Arm/Disarm (bool)/1 -> Data Type Conversion5/1
  Data Type Conversion3/1 -> Dead Zone/1
  Emergency Abort (bool)/1 -> Data Type Conversion2/1
  Data Type Conversion4/1 -> Joystick Issue (0,1)/1, Mux/4
  Yaw (%)/1 -> Mux1/3
  Pitch (%)/1 -> Mux1/2
  Roll (%)/1 -> Mux1/1
  Throttle (%)/1 -> Data Type Conversion1/1
  Mux1/1 -> Data Type Conversion3/1
  Joystick Issue (bool)/1 -> Logical Operator/1, Data Type Conversion4/1

== system QD2_MissionCtrl_Hover_FreqSwp_2021a/MISSION CONTROL QDRONE POSITION CONTROL/JOYSTICK_SPEKTRUM/Pulse Check ==
  note: For this subsystem we will count the number of new pulses. The data can be considered enabled once the count of new signals has gone beyond 2. This will enable the Initializing and conditioning subsystem.
  new : Inport
  Compare : quarc_library/Logic Operations/Compare  operator=>  output_data_type=boolean
      settings: SourceProductName=QUARC Targets
  Pulse Check : Constant  Value=2
  "pulse count " : Subsystem  TreatAsAtomicUnit=on
  signal enable : Outport  InitialOutput=0  VectorParamsAs1DForOutWhenUnconnected=off
  wires:
  Compare/1 -> signal enable/1
  Pulse Check/1 -> Compare/2
  new/1 -> "pulse count "/Trigger
  "pulse count "/1(Number of Pulses) -> Compare/1

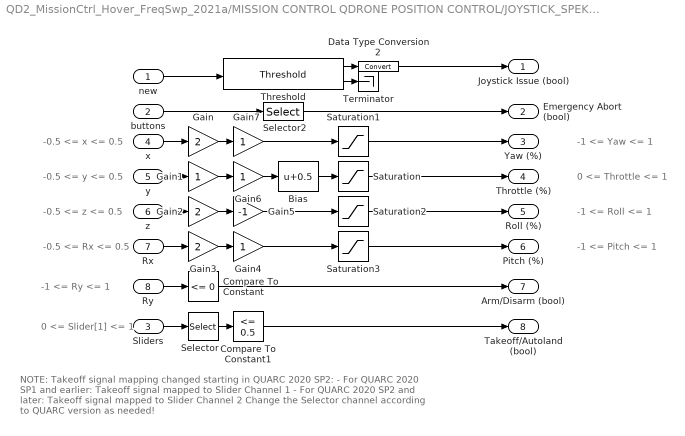
== system QD2_MissionCtrl_Hover_FreqSwp_2021a/MISSION CONTROL QDRONE POSITION CONTROL/JOYSTICK_SPEKTRUM/Spectrum DXe Mapping ==
  note: NOTE: Takeoff signal mapping changed starting in QUARC 2020 SP2:
      |
      | - For QUARC 2020 SP1 and earlier: Takeoff signal mapped to Slider Channel 1
      | - For QUARC 2020 SP2 and later: Takeoff signal mapped to Slider Channel 2
      |
      | Change the Selector channel according to QUARC version as needed!
  note: -1 <= Ry <= 1
  note: 0 <= Slider[1] <= 1
  note: -1 <= Pitch <= 1
  note: -0.5 <= Rx <= 0.5
  note: -1 <= Roll <= 1
  note: -0.5 <= z <= 0.5
  note: 0 <= Throttle <= 1
  note: -0.5 <= y <= 0.5
  note: -1 <= Yaw <= 1
  note: -0.5 <= x <= 0.5
  new : Inport
  buttons : Inport  Port=2
  Sliders : Inport  Port=3
  x : Inport  Port=4
  y : Inport  Port=5
  z : Inport  Port=6
  Rx : Inport  Port=7
  Ry : Inport  Port=8
  Bias : Bias  Bias=0.5  SaturateOnIntegerOverflow=off
  Compare To Constant : simulink/Logic and Bit Operations/Compare To Constant  relop=<=  const=0  OutDataTypeStr=boolean
  Compare To Constant1 : simulink/Logic and Bit Operations/Compare To Constant  relop=<=  const=0.5  OutDataTypeStr=boolean
  Data Type Conversion2 : DataTypeConversion  SaturateOnIntegerOverflow=off  RndMeth=Floor
  Gain : Gain  Gain=2
  Gain{1,4,6..7} (4 alike) : Gain
  Gain2 : Gain  Gain=2
  Gain3 : Gain  Gain=2
  Gain5 : Gain  Gain=-1
  Saturation : Saturate  UpperLimit=1  LowerLimit=0
  Saturation1 : Saturate  UpperLimit=1  LowerLimit=-1
  Saturation2 : Saturate  UpperLimit=1  LowerLimit=-1
  Saturation3 : Saturate  UpperLimit=1  LowerLimit=-1
  Selector : Selector  InputPortWidth=2  IndexOptions=Index vector (dialog)  Indices=[2]  OutputSizes=1
  Selector2 : Selector  InputPortWidth=32  IndexOptions=Index vector (dialog)  Indices=[1]  OutputSizes=1
  Terminator : Terminator
  Threshold : quarc_library/Discontinuities/Threshold  operator===  param_src=Specify via dialog  threshold=0  duration=1
      settings: SourceProductName=QUARC Targets
  Joystick Issue (bool) : Outport  VectorParamsAs1DForOutWhenUnconnected=off
  Emergency Abort (bool) : Outport  Port=2  VectorParamsAs1DForOutWhenUnconnected=off
  Yaw (%) : Outport  Port=3  VectorParamsAs1DForOutWhenUnconnected=off
  Throttle (%) : Outport  Port=4  VectorParamsAs1DForOutWhenUnconnected=off
  Roll (%) : Outport  Port=5  VectorParamsAs1DForOutWhenUnconnected=off
  Pitch (%) : Outport  Port=6  VectorParamsAs1DForOutWhenUnconnected=off
  "Arm/Disarm (bool) " : Outport  Port=7  VectorParamsAs1DForOutWhenUnconnected=off
  Takeoff/Autoland (bool) : Outport  Port=8  VectorParamsAs1DForOutWhenUnconnected=off
  wires:
  Data Type Conversion2/1 -> Joystick Issue (bool)/1
  new/1 -> Threshold/1
  Threshold/1 -> Data Type Conversion2/1
  Selector2/1 -> Emergency Abort (bool)/1
  Threshold/2 -> Terminator/1
  buttons/1 -> Selector2/1
  Compare To Constant1/1 -> Takeoff/Autoland (bool)/1
  Rx/1 -> Gain3/1
  y/1 -> Gain1/1
  Ry/1 -> Compare To Constant/1
  x/1 -> Gain/1
  z/1 -> Gain2/1
  Gain4/1 -> Saturation3/1
  Gain1/1 -> Gain6/1
  Gain2/1 -> Gain5/1
  Bias/1 -> Saturation/1
  Saturation2/1 -> Roll (%)/1
  Gain3/1 -> Gain4/1
  Gain/1 -> Gain7/1
  Saturation1/1 -> Yaw (%)/1
  Gain6/1 -> Bias/1
  Sliders/1 -> Selector/1
  Saturation/1 -> Throttle (%)/1
  Gain5/1 -> Saturation2/1
  Selector/1 -> Compare To Constant1/1
  Gain7/1 -> Saturation1/1
  Saturation3/1 -> Pitch (%)/1
  Compare To Constant/1 -> "Arm/Disarm (bool) "/1
